simulink model "CodeGenPlant"  (R2018b)
settings: Solver=FixedStepDiscrete  StartTime=0.0  StopTime=60  FixedStep=MdlTS  RelTol=1e-3  EnableMultiTasking=on
settings Model: DataDictionary=CodeGenPlantData.sldd  Creator=BRAUL  LastModifiedBy=BRAUL
settings OptimizationCC: DefaultParameterBehavior=Inlined  UseFloatMulNetSlope=on  UseSpecifiedMinMax=on  InlineInvariantSignals=on  PassReuseOutputArgsAs=Individual arguments  ZeroExternalMemoryAtStartup=off  ZeroInternalMemoryAtStartup=off  NoFixptDivByZeroProtection=on  EfficientFloat2IntCast=on  LifeSpan=inf  MaxStackSize=64  OptimizeBlockOrder=speed  DifferentSizesBufferReuse=on
settings DebuggingCC: MergeDetectMultiDrivingBlocksExec=none  ParameterTunabilityLossMsg=error
settings HardwareCC: ProdBitPerPointer=32  ProdBitPerSizeT=32  ProdBitPerPtrDiffT=32  ProdLargestAtomicInteger=Long  ProdLargestAtomicFloat=Double  ProdWordSize=32  ProdLongLongMode=on  ProdHWDeviceType=ARM Compatible->ARM Cortex
settings ModelReferenceCC: ModelReferenceNumInstancesAllowed=Single  PropagateSignalLabelsOutOfModel=off
settings SFSimCC: MATLABDynamicMemAlloc=off
settings RTWCC: SystemTargetFile=ert.tlc  HardwareBoard=STM32 Nucleo F411RE  GenCodeOnly=on  TemplateMakefile=ert_default_tmf  GenerateReport=on  Toolchain=GNU Tools for ARM Embedded Processors  BuildConfiguration=Faster Runs  IncludeHyperlinkInReport=on  LaunchReport=on  CodeExecutionProfiling=on  GenerateTraceInfo=on  GenerateTraceReport=on  GenerateTraceReportSl=on  GenerateTraceReportSf=on  GenerateTraceReportEml=on
settings CodeAppCC: ForceParamTrailComments=on  IgnoreCustomStorageClasses=off  OperatorAnnotations=on  SimulinkDataObjDesc=on  SFDataObjDesc=on  InsertBlockDesc=on
settings ERTTargetCC: CombineSignalStateStructs=on  SuppressErrorStatus=on  SupportNonFinite=off  SupportComplex=off

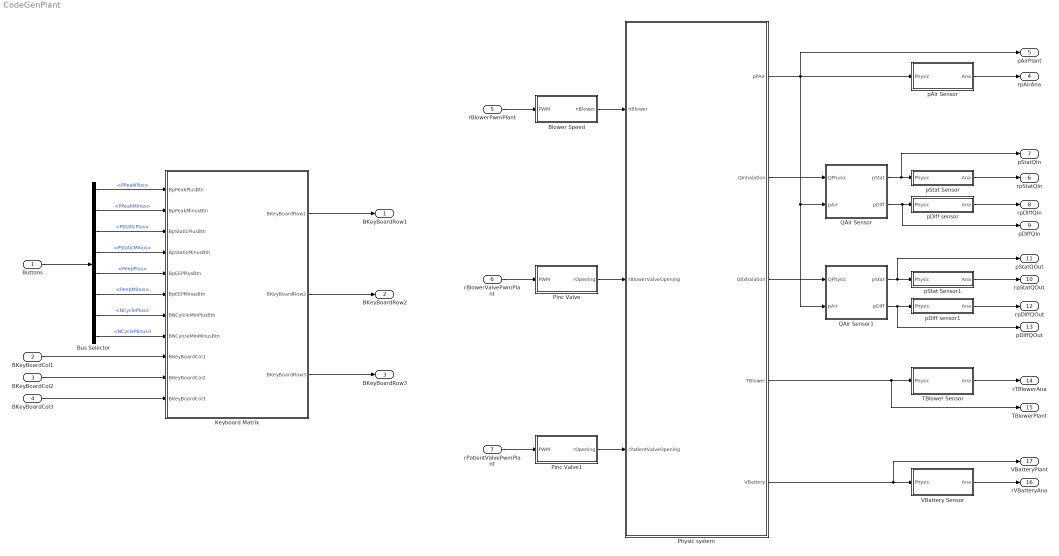
== system CodeGenPlant ==
  Buttons : Inport  OutDataTypeStr=Bus: UserButtons
  BKeyBoardCol1 : Inport  Port=2  OutDataTypeStr=boolean  PortDimensions=1
  BKeyBoardCol2 : Inport  Port=3  OutDataTypeStr=boolean  PortDimensions=1
  BKeyBoardCol3 : Inport  Port=4  OutDataTypeStr=boolean  PortDimensions=1
  rBlowerPwmPlant : Inport  Port=5
  rBlowerValvePwmPlant : Inport  Port=6
  rPatientValvePwmPlant : Inport  Port=7
  Blower Speed : Subsystem
  Bus Selector : BusSelector  OutputSignals=PPeakPlus,PPeakMinus,PStaticPlus,PStaticMinus,PeepPlus,PeepMinus,NCyclePlus,NCycleMinus
  Keyboard Matrix : Subsystem
  Physic system : Subsystem
  Pinc Valve : Subsystem
  Pinc Valve1 : Subsystem
  QAir Sensor : Subsystem
  QAir Sensor1 : Subsystem
  TBlower Sensor : Subsystem
  VBattery Sensor : Subsystem
  pAir Sensor : Subsystem
  pDiff sensor : Subsystem
  pDiff sensor1 : Subsystem
  pStat Sensor : Subsystem
  pStat Sensor1 : Subsystem
  BKeyBoardRow1 : Outport  OutDataTypeStr=boolean  PortDimensions=1
  BKeyBoardRow2 : Outport  Port=2  OutDataTypeStr=boolean  PortDimensions=1
  BKeyBoardRow3 : Outport  Port=3  OutDataTypeStr=boolean  PortDimensions=1
  rpAirAna : Outport  Port=4
  pAirPlant : Outport  Port=5
  rpStatQIn : Outport  Port=6
  pStatQIn : Outport  Port=7
  rpDiffQIn : Outport  Port=8
  pDiffQIn : Outport  Port=9
  rpStatQOut : Outport  Port=10
  pStatQOut : Outport  Port=11
  rpDiffQOut : Outport  Port=12
  pDiffQOut : Outport  Port=13
  rTBlowerAna : Outport  Port=14
  TBlowerPlant : Outport  Port=15
  rVBatteryAna : Outport  Port=16
  VBatteryPlant : Outport  Port=17
  wires:
  pAir Sensor/1(Ana) -> rpAirAna/1
  Physic system/1(pPAir) -> pAirPlant/1, pAir Sensor/1(Physic), QAir Sensor1/2(pAir), QAir Sensor/2(pAir)
  rBlowerPwmPlant/1 -> Blower Speed/1(PWM)
  rBlowerValvePwmPlant/1 -> Pinc Valve/1(PWM)
  Pinc Valve/1(rOpening) -> Physic system/2(rBlowerValveOpening)
  rPatientValvePwmPlant/1 -> Pinc Valve1/1(PWM)
  Pinc Valve1/1(rOpening) -> Physic system/3(rPatientValveOpening)
  Blower Speed/1(nBlower) -> Physic system/1(nBlower)
  TBlower Sensor/1(Ana) -> rTBlowerAna/1
  VBattery Sensor/1(Ana) -> rVBatteryAna/1
  Physic system/5(VBattery) -> VBatteryPlant/1, VBattery Sensor/1(Physic)
  Physic system/4(TBlower) -> TBlowerPlant/1, TBlower Sensor/1(Physic)
  Keyboard Matrix/2(BKeyBoardRow2) -> BKeyBoardRow2/1
  Keyboard Matrix/1(BKeyBoardRow1) -> BKeyBoardRow1/1
  Keyboard Matrix/3(BKeyBoardRow3) -> BKeyBoardRow3/1
  BKeyBoardCol1/1 -> Keyboard Matrix/9(BKeyBoardCol1)
  BKeyBoardCol2/1 -> Keyboard Matrix/10(BKeyBoardCol2)
  BKeyBoardCol3/1 -> Keyboard Matrix/11(BKeyBoardCol3)
  Buttons/1 -> Bus Selector/1
  Bus Selector/1 -> Keyboard Matrix/1(BpPeakPlusBtn)  "<PPeakPlus>"
  Bus Selector/2 -> Keyboard Matrix/2(BpPeakMinusBtn)  "<PPeakMinus>"
  Bus Selector/3 -> Keyboard Matrix/3(BpStaticPlusBtn)  "<PStaticPlus>"
  Bus Selector/4 -> Keyboard Matrix/4(BpStaticMinusBtn)  "<PStaticMinus>"
  Bus Selector/5 -> Keyboard Matrix/5(BpEEPPlusBtn)  "<PeepPlus>"
  Bus Selector/6 -> Keyboard Matrix/6(BpEEPMinusBtn)  "<PeepMinus>"
  Bus Selector/7 -> Keyboard Matrix/7(BNCylcleMinPlusBtn)  "<NCyclePlus>"
  Bus Selector/8 -> Keyboard Matrix/8(BNCylcleMinMinusBtn)  "<NCycleMinus>"
  Physic system/2(QInhalation) -> QAir Sensor/1(QPhysic)
  Physic system/3(QExhalation) -> QAir Sensor1/1(QPhysic)
  QAir Sensor/1(pStat) -> pStat Sensor/1(Physic), pStatQIn/1
  QAir Sensor/2(pDiff) -> pDiffQIn/1, pDiff sensor/1(Physic)
  QAir Sensor1/1(pStat) -> pStat Sensor1/1(Physic), pStatQOut/1
  QAir Sensor1/2(pDiff) -> pDiff sensor1/1(Physic), pDiffQOut/1
  pStat Sensor/1(Ana) -> rpStatQIn/1
  pDiff sensor/1(Ana) -> rpDiffQIn/1
  pStat Sensor1/1(Ana) -> rpStatQOut/1
  pDiff sensor1/1(Ana) -> rpDiffQOut/1

== system CodeGenPlant/Blower Speed ==
  note: % 100% PWM = 55 krpm
      | gain = 55e3/100
  PWM : Inport  OutDataTypeStr=single
  Gain : Gain  Gain=55e3/100
  nBlower : Outport  OutDataTypeStr=single
  wires:
  PWM/1 -> Gain/1
  Gain/1 -> nBlower/1

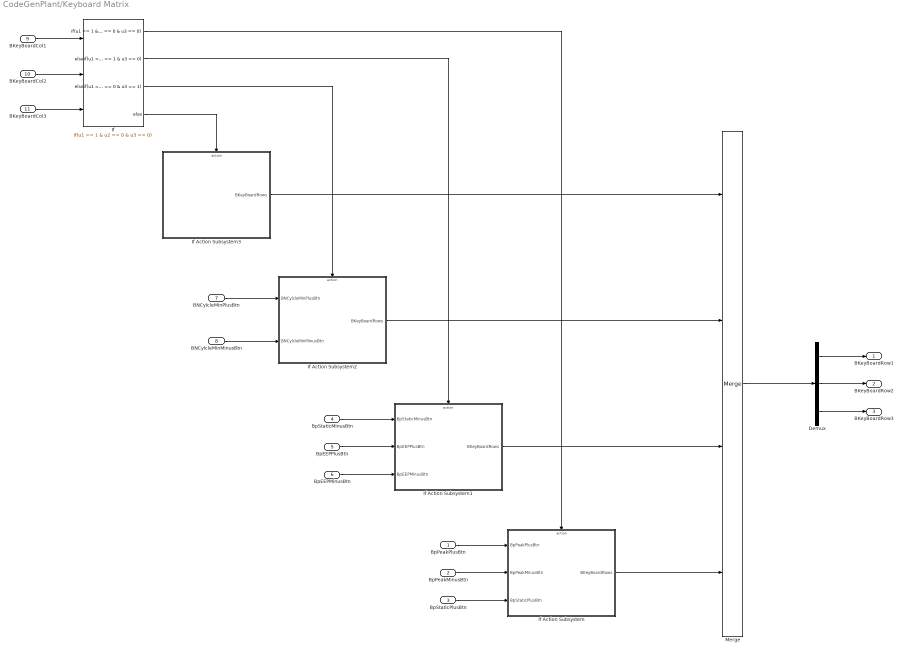
== system CodeGenPlant/Keyboard Matrix ==
  BpPeakPlusBtn : Inport  OutDataTypeStr=boolean  PortDimensions=1
  BpPeakMinusBtn : Inport  Port=2  OutDataTypeStr=boolean  PortDimensions=1
  BpStaticPlusBtn : Inport  Port=3  OutDataTypeStr=boolean  PortDimensions=1
  BpStaticMinusBtn : Inport  Port=4  OutDataTypeStr=boolean  PortDimensions=1
  BpEEPPlusBtn : Inport  Port=5  OutDataTypeStr=boolean  PortDimensions=1
  BpEEPMinusBtn : Inport  Port=6  OutDataTypeStr=boolean  PortDimensions=1
  BNCylcleMinPlusBtn : Inport  Port=7  OutDataTypeStr=boolean  PortDimensions=1
  BNCylcleMinMinusBtn : Inport  Port=8  OutDataTypeStr=boolean  PortDimensions=1
  BKeyBoardCol1 : Inport  Port=9  OutDataTypeStr=boolean  PortDimensions=1
  BKeyBoardCol2 : Inport  Port=10  OutDataTypeStr=boolean  PortDimensions=1
  BKeyBoardCol3 : Inport  Port=11  OutDataTypeStr=boolean  PortDimensions=1
  Demux : Demux  Outputs=3
  If : If  NumInputs=3  IfExpression=u1 == 1 & u2 == 0 & u3 == 0  ElseIfExpressions=u1 == 0 & u2 == 1 & u3 == 0, u1 == 0 & u2 == 0 & u3 == 1
  If Action Subsystem : Subsystem  TreatAsAtomicUnit=on
  If Action Subsystem1 : Subsystem  TreatAsAtomicUnit=on
  If Action Subsystem2 : Subsystem  TreatAsAtomicUnit=on
  If Action Subsystem3 : Subsystem  TreatAsAtomicUnit=on
  Merge : Merge  Inputs=4  InitialOutput=[0 0 0]
  BKeyBoardRow1 : Outport  OutDataTypeStr=boolean  PortDimensions=1
  BKeyBoardRow2 : Outport  Port=2  OutDataTypeStr=boolean  PortDimensions=1
  BKeyBoardRow3 : Outport  Port=3  OutDataTypeStr=boolean  PortDimensions=1
  wires:
  BKeyBoardCol2/1 -> If/2
  BKeyBoardCol1/1 -> If/1
  BKeyBoardCol3/1 -> If/3
  BNCylcleMinMinusBtn/1 -> If Action Subsystem2/2(BNCylcleMinMinusBtn)
  BNCylcleMinPlusBtn/1 -> If Action Subsystem2/1(BNCylcleMinPlusBtn)
  BpStaticMinusBtn/1 -> If Action Subsystem1/1(BpStaticMinusBtn)
  BpEEPPlusBtn/1 -> If Action Subsystem1/2(BpEEPPlusBtn)
  BpEEPMinusBtn/1 -> If Action Subsystem1/3(BpEEPMinusBtn)
  BpPeakPlusBtn/1 -> If Action Subsystem/1(BpPeakPlusBtn)
  BpPeakMinusBtn/1 -> If Action Subsystem/2(BpPeakMinusBtn)
  BpStaticPlusBtn/1 -> If Action Subsystem/3(BpStaticPlusBtn)
  If/4 -> If Action Subsystem3/Action
  If/3 -> If Action Subsystem2/Action
  If/2 -> If Action Subsystem1/Action
  If/1 -> If Action Subsystem/Action
  If Action Subsystem1/1(BKeyBoardRows) -> Merge/3
  Merge/1 -> Demux/1
  Demux/1 -> BKeyBoardRow1/1
  Demux/2 -> BKeyBoardRow2/1
  Demux/3 -> BKeyBoardRow3/1
  If Action Subsystem/1(BKeyBoardRows) -> Merge/4
  If Action Subsystem3/1(BKeyBoardRows) -> Merge/1
  If Action Subsystem2/1(BKeyBoardRows) -> Merge/2

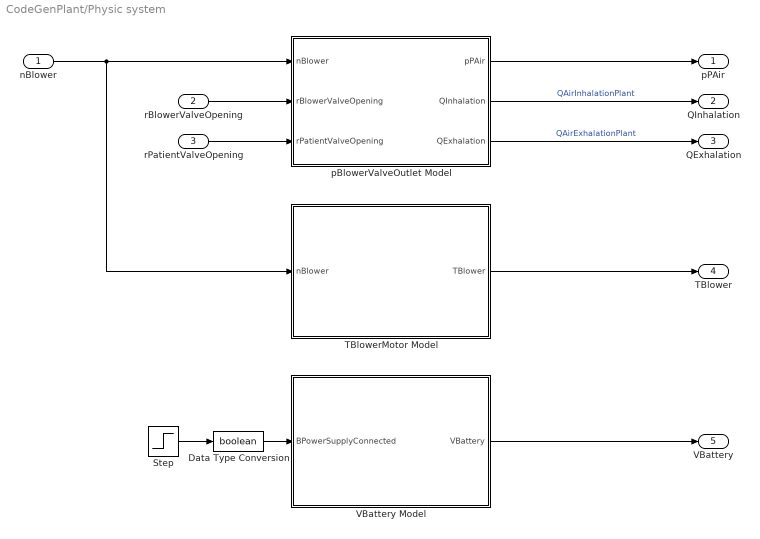
== system CodeGenPlant/Physic system ==
  nBlower : Inport
  rBlowerValveOpening : Inport  Port=2
  rPatientValveOpening : Inport  Port=3
  Data Type Conversion : DataTypeConversion  OutDataTypeStr=boolean
  Step : Step  Time=45  Before=1  After=0
  TBlowerMotor Model : Subsystem
  VBattery Model : Subsystem
  pBlowerValveOutlet Model : Subsystem
  pPAir : Outport  OutDataTypeStr=single
  QInhalation : Outport  Port=2  OutDataTypeStr=single
  QExhalation : Outport  Port=3  OutDataTypeStr=single
  TBlower : Outport  Port=4  OutDataTypeStr=single
  VBattery : Outport  Port=5  OutDataTypeStr=single
  wires:
  rBlowerValveOpening/1 -> pBlowerValveOutlet Model/2(rBlowerValveOpening)
  rPatientValveOpening/1 -> pBlowerValveOutlet Model/3(rPatientValveOpening)
  pBlowerValveOutlet Model/1(pPAir) -> pPAir/1
  TBlowerMotor Model/1(TBlower) -> TBlower/1
  VBattery Model/1(VBattery) -> VBattery/1
  nBlower/1 -> TBlowerMotor Model/1(nBlower), pBlowerValveOutlet Model/1(nBlower)
  Data Type Conversion/1 -> VBattery Model/1(BPowerSupplyConnected)
  Step/1 -> Data Type Conversion/1
  pBlowerValveOutlet Model/2(QInhalation) -> QInhalation/1  "QAirInhalationPlant"
  pBlowerValveOutlet Model/3(QExhalation) -> QExhalation/1  "QAirExhalationPlant"

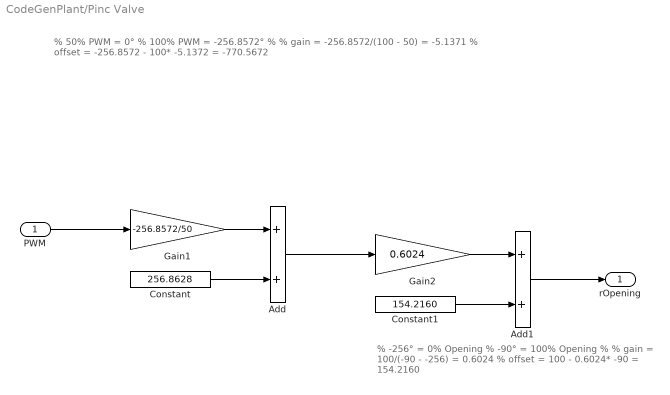
== system CodeGenPlant/Pinc Valve ==
  note: % 50% PWM = 0°
      | % 100% PWM = -256.8572°
      | %
      | % gain = -256.8572/(100 - 50) = -5.1371
      | % offset = -256.8572 - 100* -5.1372 = -770.5672
  note: % -256° = 0% Opening
      | % -90° = 100% Opening
      | %
      | % gain = 100/(-90 - -256) = 0.6024
      | % offset = 100 - 0.6024* -90 = 154.2160
  PWM : Inport  OutDataTypeStr=single
  Add : Sum
  Add1 : Sum
  Constant : Constant  Value=256.8628  OutDataTypeStr=single
  Constant1 : Constant  Value=154.2160  OutDataTypeStr=single
  Gain1 : Gain  Gain=-256.8572/50
  Gain2 : Gain  Gain=0.6024
  rOpening : Outport  OutDataTypeStr=single
  wires:
  Add/1 -> Gain2/1
  Gain1/1 -> Add/1
  Constant/1 -> Add/2
  PWM/1 -> Gain1/1
  Constant1/1 -> Add1/2
  Gain2/1 -> Add1/1
  Add1/1 -> rOpening/1

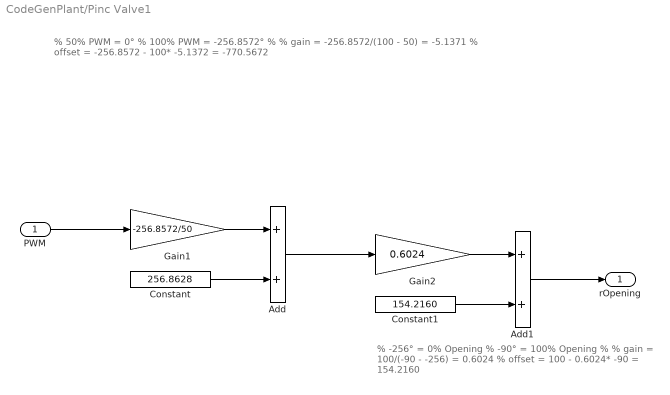
== system CodeGenPlant/Pinc Valve1 ==
  note: % -256° = 0% Opening
      | % -90° = 100% Opening
      | %
      | % gain = 100/(-90 - -256) = 0.6024
      | % offset = 100 - 0.6024* -90 = 154.2160
  note: % 50% PWM = 0°
      | % 100% PWM = -256.8572°
      | %
      | % gain = -256.8572/(100 - 50) = -5.1371
      | % offset = -256.8572 - 100* -5.1372 = -770.5672
  PWM : Inport  OutDataTypeStr=single
  Add : Sum
  Add1 : Sum
  Constant : Constant  Value=256.8628  OutDataTypeStr=single
  Constant1 : Constant  Value=154.2160  OutDataTypeStr=single
  Gain1 : Gain  Gain=-256.8572/50
  Gain2 : Gain  Gain=0.6024
  rOpening : Outport  OutDataTypeStr=single
  wires:
  Add1/1 -> rOpening/1
  Gain2/1 -> Add1/1
  Constant1/1 -> Add1/2
  PWM/1 -> Gain1/1
  Constant/1 -> Add/2
  Gain1/1 -> Add/1
  Add/1 -> Gain2/1

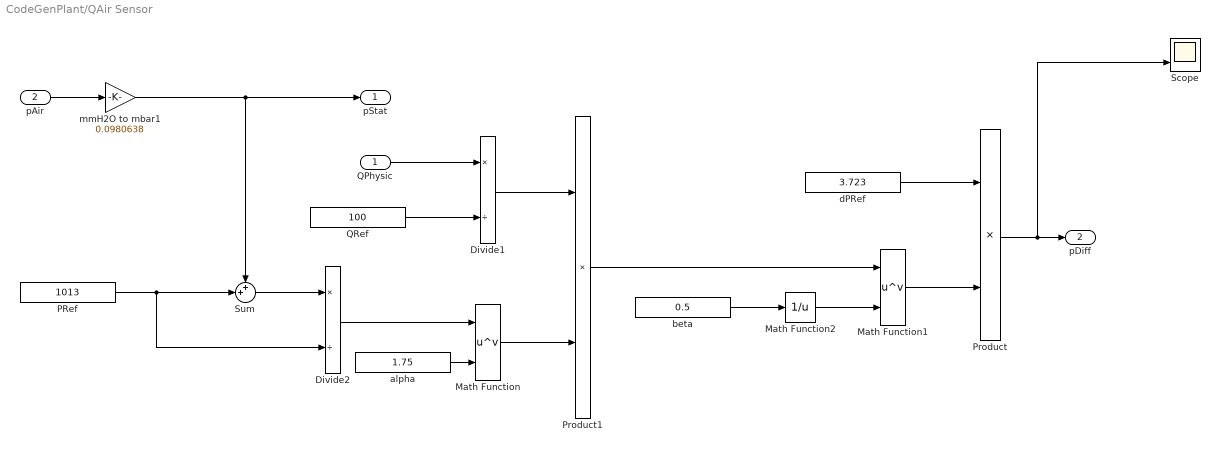
== system CodeGenPlant/QAir Sensor ==
  QPhysic : Inport
  pAir : Inport  Port=2
  Divide1 : Product  Inputs=*/
  Divide2 : Product  Inputs=*/
  Math Function : Math  Operator=pow  SaturateOnIntegerOverflow=on
  Math Function1 : Math  Operator=pow  SaturateOnIntegerOverflow=on
  Math Function2 : Math  Operator=reciprocal  SaturateOnIntegerOverflow=on
  PRef : Constant  Value=1013  OutDataTypeStr=single
  Product : Product
  Product1 : Product
  QRef : Constant  Value=100  OutDataTypeStr=single
  Scope : Scope  NumInputPorts=2
  Sum : Sum  Inputs=++|
  alpha : Constant  Value=1.75  OutDataTypeStr=single
  beta : Constant  Value=0.5  OutDataTypeStr=single
  dPRef : Constant  Value=3.723  OutDataTypeStr=single
  mmH2O to mbar1 : Gain  Gain=0.0980638
  pStat : Outport
  pDiff : Outport  Port=2
  wires:
  dPRef/1 -> Product/1
  Divide1/1 -> Product1/1
  QPhysic/1 -> Divide1/1
  QRef/1 -> Divide1/2
  PRef/1 -> Divide2/2, Sum/2
  Divide2/1 -> Math Function/1
  alpha/1 -> Math Function/2
  Math Function/1 -> Product1/2
  beta/1 -> Math Function2/1
  Math Function2/1 -> Math Function1/2
  Product1/1 -> Math Function1/1
  Math Function1/1 -> Product/2
  Product/1 -> Scope/2, pDiff/1
  pAir/1 -> mmH2O to mbar1/1
  mmH2O to mbar1/1 -> pStat/1, Sum/1
  Sum/1 -> Divide2/1

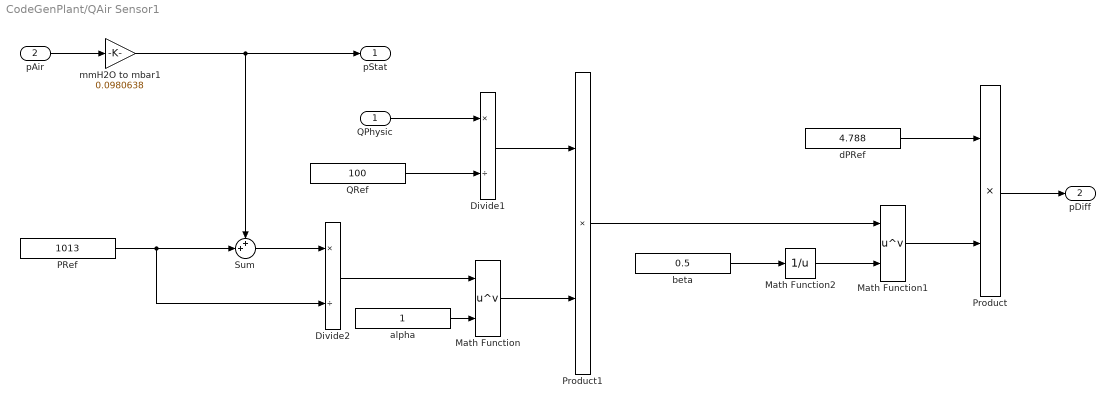
== system CodeGenPlant/QAir Sensor1 ==
  QPhysic : Inport
  pAir : Inport  Port=2
  Divide1 : Product  Inputs=*/
  Divide2 : Product  Inputs=*/
  Math Function : Math  Operator=pow  SaturateOnIntegerOverflow=on
  Math Function1 : Math  Operator=pow  SaturateOnIntegerOverflow=on
  Math Function2 : Math  Operator=reciprocal  SaturateOnIntegerOverflow=on
  PRef : Constant  Value=1013  OutDataTypeStr=single
  Product : Product
  Product1 : Product
  QRef : Constant  Value=100  OutDataTypeStr=single
  Sum : Sum  Inputs=++|
  alpha : Constant  OutDataTypeStr=single
  beta : Constant  Value=0.5  OutDataTypeStr=single
  dPRef : Constant  Value=4.788  OutDataTypeStr=single
  mmH2O to mbar1 : Gain  Gain=0.0980638
  pStat : Outport
  pDiff : Outport  Port=2
  wires:
  Sum/1 -> Divide2/1
  mmH2O to mbar1/1 -> Sum/1, pStat/1
  pAir/1 -> mmH2O to mbar1/1
  Product/1 -> pDiff/1
  Math Function1/1 -> Product/2
  Product1/1 -> Math Function1/1
  Math Function2/1 -> Math Function1/2
  beta/1 -> Math Function2/1
  Math Function/1 -> Product1/2
  alpha/1 -> Math Function/2
  Divide2/1 -> Math Function/1
  PRef/1 -> Sum/2, Divide2/2
  QRef/1 -> Divide1/2
  QPhysic/1 -> Divide1/1
  Divide1/1 -> Product1/1
  dPRef/1 -> Product/1

== system CodeGenPlant/TBlower Sensor ==
  Physic : Inport
  1-D Lookup Table : Lookup_n-D  NumberOfTableDimensions=1  BreakpointsForDimension1=[-20 -4 4 19.5 78.5 96 110 125]  Table=[3200 3070 2966 2670 1000 666 476 333]  InternalRulePriority=Speed  RndMeth=Simplest  InputSameDT=on
  Constant : Constant  Value=3300  OutDataTypeStr=single
  Divide : Product  Inputs=*/
  Saturation : Saturate  UpperLimit=1  LowerLimit=0
  Ana : Outport
  wires:
  Saturation/1 -> Ana/1
  Divide/1 -> Saturation/1
  Constant/1 -> Divide/2
  Physic/1 -> 1-D Lookup Table/1
  1-D Lookup Table/1 -> Divide/1  "VTBlowerAnaPlant"

== system CodeGenPlant/VBattery Sensor ==
  note: % Physic max = 27.6 V
      | % Physic min = 0 V
      | % Elec min = 0 mV
      | % Elec max = 3000 mV
      |
      | % => Gain = 3000/27.6 = 108.695
      | % => Offset = 0
  Physic : Inport
  Constant : Constant  Value=3300  OutDataTypeStr=single
  Divide : Product  Inputs=*/
  Gain : Gain  Gain=3000/27.6
  Saturation : Saturate  UpperLimit=1  LowerLimit=0
  Ana : Outport
  wires:
  Physic/1 -> Gain/1
  Constant/1 -> Divide/2
  Divide/1 -> Saturation/1
  Saturation/1 -> Ana/1
  Gain/1 -> Divide/1

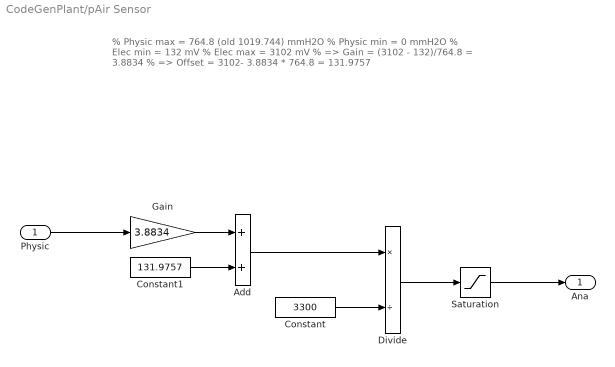
== system CodeGenPlant/pAir Sensor ==
  note: % Physic max = 764.8 (old 1019.744) mmH2O
      | % Physic min = 0 mmH2O
      | % Elec min = 132 mV
      | % Elec max = 3102 mV
      |
      | % => Gain = (3102 - 132)/764.8 = 3.8834
      | % => Offset = 3102- 3.8834 * 764.8 = 131.9757
  Physic : Inport
  Add : Sum
  Constant : Constant  Value=3300  OutDataTypeStr=single
  Constant1 : Constant  Value=131.9757  OutDataTypeStr=single
  Divide : Product  Inputs=*/
  Gain : Gain  Gain=3.8834
  Saturation : Saturate  UpperLimit=1  LowerLimit=0
  Ana : Outport
  wires:
  Physic/1 -> Gain/1
  Constant/1 -> Divide/2
  Divide/1 -> Saturation/1
  Saturation/1 -> Ana/1
  Add/1 -> Divide/1
  Constant1/1 -> Add/2
  Gain/1 -> Add/1

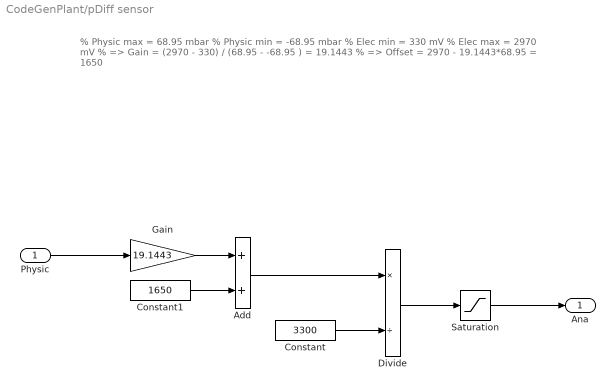
== system CodeGenPlant/pDiff sensor ==
  note: % Physic max = 68.95 mbar
      | % Physic min = -68.95 mbar
      | % Elec min = 330 mV
      | % Elec max = 2970 mV
      |
      | % => Gain = (2970 - 330) / (68.95 - -68.95 ) = 19.1443
      | % => Offset = 2970 - 19.1443*68.95 = 1650
  Physic : Inport
  Add : Sum
  Constant : Constant  Value=3300  OutDataTypeStr=single
  Constant1 : Constant  Value=1650  OutDataTypeStr=single
  Divide : Product  Inputs=*/
  Gain : Gain  Gain=19.1443
  Saturation : Saturate  UpperLimit=1  LowerLimit=0
  Ana : Outport
  wires:
  Physic/1 -> Gain/1
  Constant/1 -> Divide/2
  Divide/1 -> Saturation/1
  Saturation/1 -> Ana/1
  Add/1 -> Divide/1
  Constant1/1 -> Add/2
  Gain/1 -> Add/1

== system CodeGenPlant/pDiff sensor1 ==
  note: % Physic max = 68.95 mbar
      | % Physic min = -68.95 mbar
      | % Elec min = 330 mV
      | % Elec max = 2970 mV
      |
      | % => Gain = (2970 - 330) / (68.95 - -68.95 ) = 19.1443
      | % => Offset = 2970 - 19.1443*68.95 = 1650
  Physic : Inport
  Add : Sum
  Constant : Constant  Value=3300  OutDataTypeStr=single
  Constant1 : Constant  Value=1650  OutDataTypeStr=single
  Divide : Product  Inputs=*/
  Gain : Gain  Gain=19.1443
  Saturation : Saturate  UpperLimit=1  LowerLimit=0
  Ana : Outport
  wires:
  Gain/1 -> Add/1
  Constant1/1 -> Add/2
  Add/1 -> Divide/1
  Saturation/1 -> Ana/1
  Divide/1 -> Saturation/1
  Constant/1 -> Divide/2
  Physic/1 -> Gain/1

== system CodeGenPlant/pStat Sensor ==
  note: % Physic max = 100 mbar
      | % Physic min = 0 mbar
      | % Elec min = 132 mV
      | % Elec max = 3102 mV
      |
      | % => Gain = (3102 - 132)/100 = 29.7000
      | % => Offset = 3102- 29.7*100 = 132
  Physic : Inport
  Add : Sum
  Constant : Constant  Value=3300  OutDataTypeStr=single
  Constant1 : Constant  Value=132  OutDataTypeStr=single
  Divide : Product  Inputs=*/
  Gain : Gain  Gain=29.7
  Saturation : Saturate  UpperLimit=1  LowerLimit=0
  Ana : Outport
  wires:
  Gain/1 -> Add/1
  Constant1/1 -> Add/2
  Add/1 -> Divide/1
  Saturation/1 -> Ana/1
  Divide/1 -> Saturation/1
  Constant/1 -> Divide/2
  Physic/1 -> Gain/1

== system CodeGenPlant/pStat Sensor1 ==
  note: % Physic max = 100 mbar
      | % Physic min = 0 mbar
      | % Elec min = 132 mV
      | % Elec max = 3102 mV
      |
      | % => Gain = (3102 - 132)/100 = 29.7000
      | % => Offset = 3102- 29.7*100 = 132
  Physic : Inport
  Add : Sum
  Constant : Constant  Value=3300  OutDataTypeStr=single
  Constant1 : Constant  Value=132  OutDataTypeStr=single
  Divide : Product  Inputs=*/
  Gain : Gain  Gain=29.7
  Saturation : Saturate  UpperLimit=1  LowerLimit=0
  Ana : Outport
  wires:
  Physic/1 -> Gain/1
  Constant/1 -> Divide/2
  Divide/1 -> Saturation/1
  Saturation/1 -> Ana/1
  Add/1 -> Divide/1
  Constant1/1 -> Add/2
  Gain/1 -> Add/1

== system CodeGenPlant/Keyboard Matrix/If Action Subsystem ==
  BpPeakPlusBtn : Inport  OutDataTypeStr=boolean  PortDimensions=1
  BpPeakMinusBtn : Inport  Port=2  OutDataTypeStr=boolean  PortDimensions=1
  BpStaticPlusBtn : Inport  Port=3  OutDataTypeStr=boolean  PortDimensions=1
  Action Port : ActionPort  ActionType=then
  Mux : Mux  Inputs=3
  BKeyBoardRows : Outport  OutDataTypeStr=boolean  PortDimensions=3  InitialOutput=[0 0 0]
  wires:
  BpPeakPlusBtn/1 -> Mux/1
  BpPeakMinusBtn/1 -> Mux/2
  BpStaticPlusBtn/1 -> Mux/3
  Mux/1 -> BKeyBoardRows/1

== system CodeGenPlant/Keyboard Matrix/If Action Subsystem1 ==
  BpStaticMinusBtn : Inport  OutDataTypeStr=boolean  PortDimensions=1
  BpEEPPlusBtn : Inport  Port=2  OutDataTypeStr=boolean  PortDimensions=1
  BpEEPMinusBtn : Inport  Port=3  OutDataTypeStr=boolean  PortDimensions=1
  Action Port : ActionPort  ActionType=elseif
  Mux : Mux  Inputs=3
  BKeyBoardRows : Outport  OutDataTypeStr=boolean  PortDimensions=3  InitialOutput=[0 0 0]
  wires:
  BpStaticMinusBtn/1 -> Mux/1
  Mux/1 -> BKeyBoardRows/1
  BpEEPPlusBtn/1 -> Mux/2
  BpEEPMinusBtn/1 -> Mux/3

== system CodeGenPlant/Keyboard Matrix/If Action Subsystem2 ==
  BNCylcleMinPlusBtn : Inport  OutDataTypeStr=boolean  PortDimensions=1
  BNCylcleMinMinusBtn : Inport  Port=2  OutDataTypeStr=boolean  PortDimensions=1
  Action Port : ActionPort  ActionType=elseif
  Constant : Constant  Value=false  OutDataTypeStr=boolean
  Mux : Mux  Inputs=3
  BKeyBoardRows : Outport  OutDataTypeStr=boolean  PortDimensions=3  InitialOutput=[0 0 0]
  wires:
  BNCylcleMinPlusBtn/1 -> Mux/1
  BNCylcleMinMinusBtn/1 -> Mux/2
  Mux/1 -> BKeyBoardRows/1
  Constant/1 -> Mux/3

== system CodeGenPlant/Keyboard Matrix/If Action Subsystem3 ==
  Action Port : ActionPort  ActionType=else
  Constant : Constant  Value=false  OutDataTypeStr=boolean
  Constant1 : Constant  Value=false  OutDataTypeStr=boolean
  Constant2 : Constant  Value=false  OutDataTypeStr=boolean
  Mux : Mux  Inputs=3
  BKeyBoardRows : Outport  OutDataTypeStr=boolean  PortDimensions=3  InitialOutput=[0 0 0]
  wires:
  Mux/1 -> BKeyBoardRows/1
  Constant/1 -> Mux/1
  Constant1/1 -> Mux/2
  Constant2/1 -> Mux/3

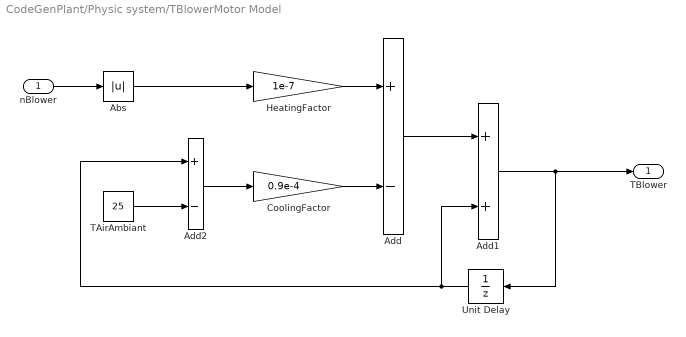
== system CodeGenPlant/Physic system/TBlowerMotor Model ==
  nBlower : Inport
  Abs : Abs
  Add : Sum  Inputs=+-
  Add1 : Sum
  Add2 : Sum  Inputs=+-
  CoolingFactor : Gain  Gain=0.9e-4
  HeatingFactor : Gain  Gain=1e-7
  TAirAmbiant : Constant  Value=25  OutDataTypeStr=single
  Unit Delay : UnitDelay  InitialCondition=25  SampleTime=-1
  TBlower : Outport  OutDataTypeStr=single
  wires:
  Unit Delay/1 -> Add1/2, Add2/1
  TAirAmbiant/1 -> Add2/2
  CoolingFactor/1 -> Add/2
  Add2/1 -> CoolingFactor/1
  Add1/1 -> TBlower/1, Unit Delay/1
  Add/1 -> Add1/1
  HeatingFactor/1 -> Add/1
  Abs/1 -> HeatingFactor/1
  nBlower/1 -> Abs/1

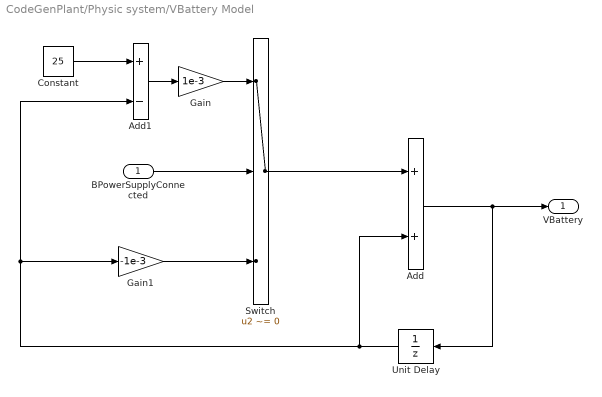
== system CodeGenPlant/Physic system/VBattery Model ==
  BPowerSupplyConnected : Inport
  Add : Sum
  Add1 : Sum  Inputs=+-
  Constant : Constant  Value=25  OutDataTypeStr=single
  Gain : Gain  Gain=1e-3
  Gain1 : Gain  Gain=-1e-3
  Switch : Switch  Criteria=u2 ~= 0
  Unit Delay : UnitDelay  InitialCondition=25  SampleTime=-1
  VBattery : Outport  OutDataTypeStr=single
  wires:
  Add/1 -> Unit Delay/1, VBattery/1
  BPowerSupplyConnected/1 -> Switch/2
  Switch/1 -> Add/1
  Add1/1 -> Gain/1
  Constant/1 -> Add1/1
  Unit Delay/1 -> Add/2, Gain1/1, Add1/2
  Gain/1 -> Switch/1
  Gain1/1 -> Switch/3

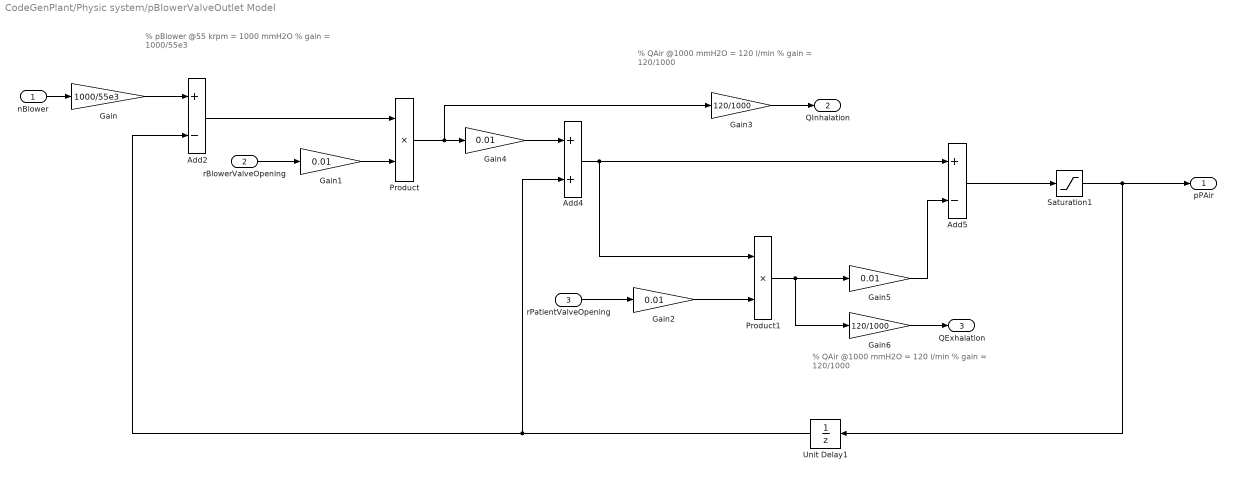
== system CodeGenPlant/Physic system/pBlowerValveOutlet Model ==
  note: % pBlower @55 krpm = 1000 mmH2O
      | % gain = 1000/55e3
  note: % QAir @1000 mmH2O = 120 l/min
      | % gain = 120/1000
  note: % QAir @1000 mmH2O = 120 l/min
      | % gain = 120/1000
  nBlower : Inport
  rBlowerValveOpening : Inport  Port=2
  rPatientValveOpening : Inport  Port=3
  Add2 : Sum  Inputs=+-
  Add4 : Sum
  Add5 : Sum  Inputs=+-
  Gain : Gain  Gain=1000/55e3
  Gain{1..2,4..5} (4 alike) : Gain  Gain=0.01
  Gain3 : Gain  Gain=120/1000
  Gain6 : Gain  Gain=120/1000
  Product : Product
  Product1 : Product
  Saturation1 : Saturate  UpperLimit=inf  LowerLimit=0
  Unit Delay1 : UnitDelay  SampleTime=-1
  pPAir : Outport  OutDataTypeStr=single
  QInhalation : Outport  Port=2  OutDataTypeStr=single
  QExhalation : Outport  Port=3  OutDataTypeStr=single
  wires:
  Unit Delay1/1 -> Add4/2, Add2/2
  Gain1/1 -> Product/2
  Add2/1 -> Product/1
  Add4/1 -> Add5/1, Product1/1
  rBlowerValveOpening/1 -> Gain1/1
  Product/1 -> Gain3/1, Gain4/1
  rPatientValveOpening/1 -> Gain2/1
  Gain4/1 -> Add4/1
  Gain/1 -> Add2/1
  Saturation1/1 -> pPAir/1, Unit Delay1/1
  Gain2/1 -> Product1/2
  nBlower/1 -> Gain/1
  Add5/1 -> Saturation1/1
  Gain3/1 -> QInhalation/1
  Gain5/1 -> Add5/2
  Product1/1 -> Gain6/1, Gain5/1
  Gain6/1 -> QExhalation/1
